simulink model "kf_test"  (R2018b)
settings: Solver=VariableStepAuto  StartTime=0.0  StopTime=60  RelTol=1e-3
values from neighbouring files (symbols this model uses):
  Rv = diag([10^-2 10^-2])    [kf_test_2.m]    (also in kf_test_3.m; lab_init_lqr.m = diag([10^-5 10^-5]))
undefined symbols (not defined in the file or in its folder): Continuous, Time
libraries: cstblocks x5, ctrlSharedLib x1
settings Model: Creator=prana  LastModifiedBy=prana

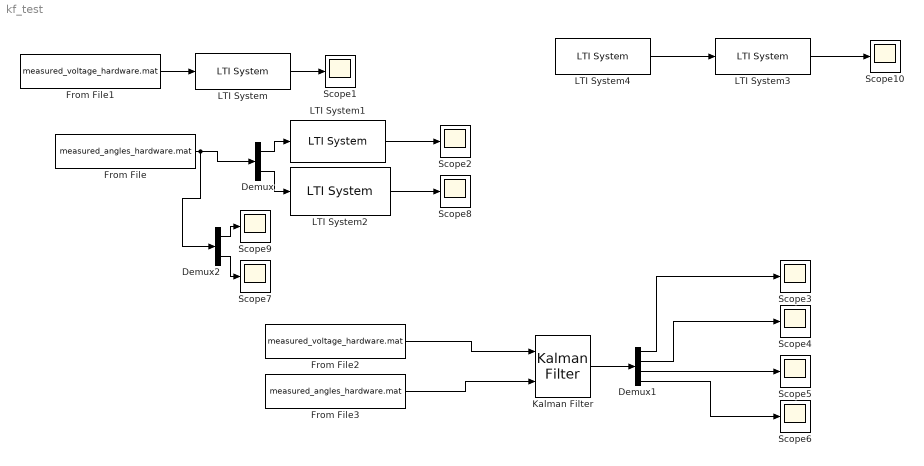
== system kf_test ==
  Demux : Demux  Outputs=2
  Demux1 : Demux
  Demux2 : Demux  Outputs=2
  From File : FromFile  FileName=measured_angles_hardware.mat  SampleTime=0
  From File1 : FromFile  FileName=measured_voltage_hardware.mat  SampleTime=0
  From File2 : FromFile  FileName=measured_voltage_hardware.mat  SampleTime=0
  From File3 : FromFile  FileName=measured_angles_hardware.mat  SampleTime=0
  Kalman Filter : ctrlSharedLib/Kalman Filter  TimeDomain=Continuous-Time  UseCurrentEstimator=on  ModelSource=LTI State-Space Variable  ModelSourceVariable=aero_sys  A=0.95  B=1  C=1  D=0  NumberOfStates=1  NumberOfInputs=1  NumberOfOutputs=1  InitialEstimateSource=Dialog  X0=0  P0=10  UseK=off  UseGH=off  NumberOfProcessNoiseInputs=1  G=1  TimeInvariantG=on  H=0  TimeInvariantH=on  Q=Rw  TimeInvariantQ=on  R=Rv  TimeInvariantR=on  N=0  TimeInvariantN=on  AddInputPort=on  AddEnablePort=off  OutputEstimatedY=off  OutputP=off  Ts=-1
      settings: SourceProductBaseCode=CT
  LTI System : cstblocks/LTI System  sys=aero_sys  IC=[]
  LTI System1 : cstblocks/LTI System  sys=Diff_LPF  IC=[]
  LTI System2 : cstblocks/LTI System  sys=Diff_LPF  IC=[]
  LTI System3 : cstblocks/LTI System  sys=aero_sys  IC=[]
  LTI System4 : cstblocks/LTI System  sys=u_hardware  IC=[]
  Scope{1..10} (10 alike) : Scope
  wires:
  From File1/1 -> LTI System/1
  LTI System/1 -> Scope1/1
  From File/1 -> Demux2/1, Demux/1
  Demux/1 -> LTI System1/1
  Demux/2 -> LTI System2/1
  LTI System1/1 -> Scope2/1
  From File2/1 -> Kalman Filter/1
  From File3/1 -> Kalman Filter/2
  Kalman Filter/1 -> Demux1/1
  Demux1/1 -> Scope3/1
  Demux1/2 -> Scope4/1
  Demux1/3 -> Scope5/1
  Demux1/4 -> Scope6/1
  LTI System2/1 -> Scope8/1
  Demux2/1 -> Scope9/1
  Demux2/2 -> Scope7/1
  LTI System3/1 -> Scope10/1
  LTI System4/1 -> LTI System3/1
